simulink model "case6"  (R2024b)
settings: Solver=FixedStepAuto  StartTime=0  StopTime=1  FixedStep=1e-7  RelTol=1e-3
values from neighbouring files (symbols this model uses):
  SG_D_1_D = 0.01056    [IEEE9_case_parameters.m]    (also in case1_parameters.m; case2_parameters.m; case3_parameters.m; case4_parameters.m)
  SG_D_1_EnableSaturation = 0    [IEEE9_case_parameters.m]    (also in case1_parameters.m; case2_parameters.m; case3_parameters.m; case4_parameters.m)
  SG_D_1_f0 = 60    [IEEE9_case_parameters.m]    (also in case1_parameters.m; case2_parameters.m; case3_parameters.m; case4_parameters.m)
  SG_D_1_H = 7.5    [IEEE9_case_parameters.m]    (also in case1_parameters.m; case2_parameters.m; case3_parameters.m; case4_parameters.m)
  SG_D_1_K_A = 20    [IEEE9_case_parameters.m]    (also in case1_parameters.m; case2_parameters.m; case3_parameters.m; case4_parameters.m)
  SG_D_1_K_E = 1.000000e+1    (= 10)    [IEEE9_case_parameters.m]    (also in case1_parameters.m; case2_parameters.m; case3_parameters.m; case4_parameters.m)
  SG_D_1_K_F = 2.363    [IEEE9_case_parameters.m]    (also in case1_parameters.m; case2_parameters.m; case3_parameters.m; case4_parameters.m)
  SG_D_1_K_s = 0.5    [IEEE9_case_parameters.m]    (also in case1_parameters.m = 5; case2_parameters.m = 5; case3_parameters.m = 5; case4_parameters.m = 5)
  SG_D_1_R_a = 0.001088    [IEEE9_case_parameters.m]    (also in case1_parameters.m; case2_parameters.m; case3_parameters.m; case4_parameters.m)
  SG_D_1_S_A = 1    [IEEE9_case_parameters.m]    (also in case1_parameters.m; case2_parameters.m; case3_parameters.m; case4_parameters.m)
  SG_D_1_S_B = 0.103    [IEEE9_case_parameters.m]    (also in case1_parameters.m; case2_parameters.m; case3_parameters.m; case4_parameters.m)
  SG_D_1_S_N = 10.659857    [IEEE9_case_parameters.m]    (also in case1_parameters.m; case2_parameters.m; case3_parameters.m; case4_parameters.m)
  SG_D_1_SpeedPara = 200    [IEEE9_case_parameters.m]    (also in case1_parameters.m; case2_parameters.m; case3_parameters.m; case4_parameters.m)
  SG_D_1_T_0 = 0.720173    [IEEE9_case_parameters.m]    (also in case1_parameters.m = 0.755522; case2_parameters.m = 0.808931; case3_parameters.m = 0.869402; case4_parameters.m = 0.729316)
  SG_D_1_T_1 = 0.3    [IEEE9_case_parameters.m]    (also in case1_parameters.m; case2_parameters.m; case3_parameters.m; case4_parameters.m)
  SG_D_1_T_2 = 0.05    [IEEE9_case_parameters.m]    (also in case1_parameters.m; case2_parameters.m; case3_parameters.m; case4_parameters.m)
  SG_D_1_T_3 = 0.02    [IEEE9_case_parameters.m]    (also in case1_parameters.m; case2_parameters.m; case3_parameters.m; case4_parameters.m)
  SG_D_1_T_4 = 0.005    [IEEE9_case_parameters.m]    (also in case1_parameters.m; case2_parameters.m; case3_parameters.m; case4_parameters.m)
  SG_D_1_T_A = 0.02    [IEEE9_case_parameters.m]    (also in case1_parameters.m; case2_parameters.m; case3_parameters.m; case4_parameters.m)
  SG_D_1_T_dd = 8.000000e+0    (= 8)    [IEEE9_case_parameters.m]    (also in case1_parameters.m; case2_parameters.m; case3_parameters.m; case4_parameters.m)
  SG_D_1_T_ddd = 0.04    [IEEE9_case_parameters.m]    (also in case1_parameters.m; case2_parameters.m; case3_parameters.m; case4_parameters.m)
  SG_D_1_T_E = 0.314    [IEEE9_case_parameters.m]    (also in case1_parameters.m; case2_parameters.m; case3_parameters.m; case4_parameters.m)
  SG_D_1_T_F = 0.35    [IEEE9_case_parameters.m]    (also in case1_parameters.m; case2_parameters.m; case3_parameters.m; case4_parameters.m)
  SG_D_1_T_qd = 0.8    [IEEE9_case_parameters.m]    (also in case1_parameters.m; case2_parameters.m; case3_parameters.m; case4_parameters.m)
  SG_D_1_T_qdd = 0.02    [IEEE9_case_parameters.m]    (also in case1_parameters.m; case2_parameters.m; case3_parameters.m; case4_parameters.m)
  SG_D_1_T_speed = 0.1    [IEEE9_case_parameters.m]    (also in case1_parameters.m = 200; case2_parameters.m = 200; case3_parameters.m = 200; case4_parameters.m = 200)
  SG_D_1_T_w = 0.5    [IEEE9_case_parameters.m]    (also in case1_parameters.m; case2_parameters.m; case3_parameters.m; case4_parameters.m)
  SG_D_1_V_ref = 1.990276    [IEEE9_case_parameters.m]    (also in case1_parameters.m = 2.042296; case2_parameters.m = 2.051388; case3_parameters.m = 2.089584; case4_parameters.m = 2.01845)
  SG_D_1_w_ref = 376.991118    [IEEE9_case_parameters.m]    (also in case1_parameters.m; case2_parameters.m; case3_parameters.m; case4_parameters.m)
  SG_D_1_wb = 6.000000e+1    (= 60)    [IEEE9_case_parameters.m]    (also in case1_parameters.m; case2_parameters.m; case3_parameters.m; case4_parameters.m)
  SG_D_1_x_d = 1.9    [IEEE9_case_parameters.m]    (also in case1_parameters.m; case2_parameters.m; case3_parameters.m; case4_parameters.m)
  SG_D_1_x_dd = 0.302    [IEEE9_case_parameters.m]    (also in case1_parameters.m; case2_parameters.m; case3_parameters.m; case4_parameters.m)
  SG_D_1_x_ddd = 0.204    [IEEE9_case_parameters.m]    (also in case1_parameters.m; case2_parameters.m; case3_parameters.m; case4_parameters.m)
  SG_D_1_x_l = 0.05    [IEEE9_case_parameters.m]    (also in case1_parameters.m; case2_parameters.m; case3_parameters.m; case4_parameters.m)
  SG_D_1_x_q = 1.3    [IEEE9_case_parameters.m]    (also in case1_parameters.m; case2_parameters.m; case3_parameters.m; case4_parameters.m)
  SG_D_1_x_qd = 0.5    [IEEE9_case_parameters.m]    (also in case1_parameters.m; case2_parameters.m; case3_parameters.m; case4_parameters.m)
  SG_D_1_x_qdd = 0.3    [IEEE9_case_parameters.m]    (also in case1_parameters.m; case2_parameters.m; case3_parameters.m; case4_parameters.m)
  SG_D_2_D = 0.02    [IEEE9_case_parameters.m]    (also in case1_parameters.m; case2_parameters.m; case3_parameters.m; case4_parameters.m)
  SG_D_2_EnableSaturation = 0    [IEEE9_case_parameters.m]    (also in case1_parameters.m; case2_parameters.m; case3_parameters.m; case4_parameters.m)
  SG_D_2_f0 = 60    [IEEE9_case_parameters.m]    (also in case1_parameters.m; case2_parameters.m; case3_parameters.m; case4_parameters.m)
  SG_D_2_H = 8.000000e+0    (= 8)    [IEEE9_case_parameters.m]    (also in case1_parameters.m; case2_parameters.m; case3_parameters.m; case4_parameters.m)
  SG_D_2_K_A = 20    [IEEE9_case_parameters.m]    (also in case1_parameters.m; case2_parameters.m; case3_parameters.m; case4_parameters.m)
  SG_D_2_K_E = 1.000000e+1    (= 10)    [IEEE9_case_parameters.m]    (also in case1_parameters.m; case2_parameters.m; case3_parameters.m; case4_parameters.m)
  SG_D_2_K_F = 2.363    [IEEE9_case_parameters.m]    (also in case1_parameters.m; case2_parameters.m; case3_parameters.m; case4_parameters.m)
  SG_D_2_K_s = 0.5    [IEEE9_case_parameters.m]    (also in case1_parameters.m = 4; case2_parameters.m = 4; case3_parameters.m = 4; case4_parameters.m = 4)
  SG_D_2_R_a = 0.001088    [IEEE9_case_parameters.m]    (also in case1_parameters.m; case2_parameters.m; case3_parameters.m; case4_parameters.m)
  SG_D_2_S_A = 1    [IEEE9_case_parameters.m]    (also in case1_parameters.m; case2_parameters.m; case3_parameters.m; case4_parameters.m)
  SG_D_2_S_B = 0.103    [IEEE9_case_parameters.m]    (also in case1_parameters.m; case2_parameters.m; case3_parameters.m; case4_parameters.m)
  SG_D_2_S_N = 10.659857    [IEEE9_case_parameters.m]    (also in case1_parameters.m; case2_parameters.m; case3_parameters.m; case4_parameters.m)
  SG_D_2_SpeedPara = 200    [IEEE9_case_parameters.m]    (also in case1_parameters.m; case2_parameters.m; case3_parameters.m; case4_parameters.m)
  SG_D_2_T_0 = 1.632913    [IEEE9_case_parameters.m]    (also in case1_parameters.m = 1.632925; case2_parameters.m = 1.632915; case3_parameters.m = 1.632914; case4_parameters.m = 1.632927)
  SG_D_2_T_1 = 0.2    [IEEE9_case_parameters.m]    (also in case1_parameters.m; case2_parameters.m; case3_parameters.m; case4_parameters.m)
  SG_D_2_T_2 = 0.05    [IEEE9_case_parameters.m]    (also in case1_parameters.m; case2_parameters.m; case3_parameters.m; case4_parameters.m)
  SG_D_2_T_3 = 0.02    [IEEE9_case_parameters.m]    (also in case1_parameters.m; case2_parameters.m; case3_parameters.m; case4_parameters.m)
  SG_D_2_T_4 = 0.005    [IEEE9_case_parameters.m]    (also in case1_parameters.m; case2_parameters.m; case3_parameters.m; case4_parameters.m)
  SG_D_2_T_A = 0.02    [IEEE9_case_parameters.m]    (also in case1_parameters.m; case2_parameters.m; case3_parameters.m; case4_parameters.m)
  SG_D_2_T_dd = 7.9    [IEEE9_case_parameters.m]    (also in case1_parameters.m; case2_parameters.m; case3_parameters.m; case4_parameters.m)
  SG_D_2_T_ddd = 0.04    [IEEE9_case_parameters.m]    (also in case1_parameters.m; case2_parameters.m; case3_parameters.m; case4_parameters.m)
  SG_D_2_T_E = 0.314    [IEEE9_case_parameters.m]    (also in case1_parameters.m; case2_parameters.m; case3_parameters.m; case4_parameters.m)
  SG_D_2_T_F = 0.35    [IEEE9_case_parameters.m]    (also in case1_parameters.m; case2_parameters.m; case3_parameters.m; case4_parameters.m)
  SG_D_2_T_qd = 0.8    [IEEE9_case_parameters.m]    (also in case1_parameters.m; case2_parameters.m; case3_parameters.m; case4_parameters.m)
  SG_D_2_T_qdd = 0.015    [IEEE9_case_parameters.m]    (also in case1_parameters.m; case2_parameters.m; case3_parameters.m; case4_parameters.m)
  SG_D_2_T_speed = 0.1    [IEEE9_case_parameters.m]    (also in case1_parameters.m = 150; case2_parameters.m = 150; case3_parameters.m = 150; case4_parameters.m = 150)
  SG_D_2_T_w = 0.35    [IEEE9_case_parameters.m]    (also in case1_parameters.m; case2_parameters.m; case3_parameters.m; case4_parameters.m)
  SG_D_2_V_ref = 2.58547    [IEEE9_case_parameters.m]    (also in case1_parameters.m = 2.597896; case2_parameters.m = 2.587136; case3_parameters.m = 2.586042; case4_parameters.m = 2.599679)
  SG_D_2_w_ref = 376.991118    [IEEE9_case_parameters.m]    (also in case1_parameters.m; case2_parameters.m; case3_parameters.m; case4_parameters.m)
  SG_D_2_wb = 6.000000e+1    (= 60)    [IEEE9_case_parameters.m]    (also in case1_parameters.m; case2_parameters.m; case3_parameters.m; case4_parameters.m)
  SG_D_2_x_d = 1.8    [IEEE9_case_parameters.m]    (also in case1_parameters.m; case2_parameters.m; case3_parameters.m; case4_parameters.m)
  SG_D_2_x_dd = 0.302    [IEEE9_case_parameters.m]    (also in case1_parameters.m; case2_parameters.m; case3_parameters.m; case4_parameters.m)
  SG_D_2_x_ddd = 0.204    [IEEE9_case_parameters.m]    (also in case1_parameters.m; case2_parameters.m; case3_parameters.m; case4_parameters.m)
  SG_D_2_x_l = 0.05    [IEEE9_case_parameters.m]    (also in case1_parameters.m; case2_parameters.m; case3_parameters.m; case4_parameters.m)
  SG_D_2_x_q = 1.25    [IEEE9_case_parameters.m]    (also in case1_parameters.m; case2_parameters.m; case3_parameters.m; case4_parameters.m)
  SG_D_2_x_qd = 0.5    [IEEE9_case_parameters.m]    (also in case1_parameters.m; case2_parameters.m; case3_parameters.m; case4_parameters.m)
  SG_D_2_x_qdd = 0.3    [IEEE9_case_parameters.m]    (also in case1_parameters.m; case2_parameters.m; case3_parameters.m; case4_parameters.m)
  SG_D_3_D = 0.02    [IEEE9_case_parameters.m]    (also in case1_parameters.m; case2_parameters.m; case3_parameters.m; case4_parameters.m)
  SG_D_3_EnableSaturation = 0    [IEEE9_case_parameters.m]    (also in case1_parameters.m; case2_parameters.m; case3_parameters.m; case4_parameters.m)
  SG_D_3_f0 = 60    [IEEE9_case_parameters.m]    (also in case1_parameters.m; case2_parameters.m; case3_parameters.m; case4_parameters.m)
  SG_D_3_H = 7.7    [IEEE9_case_parameters.m]    (also in case1_parameters.m; case2_parameters.m; case3_parameters.m; case4_parameters.m)
  SG_D_3_K_A = 20    [IEEE9_case_parameters.m]    (also in case1_parameters.m; case2_parameters.m; case3_parameters.m; case4_parameters.m)
  SG_D_3_K_E = 1.000000e+1    (= 10)    [IEEE9_case_parameters.m]    (also in case1_parameters.m; case2_parameters.m; case3_parameters.m; case4_parameters.m)
  SG_D_3_K_F = 2.363    [IEEE9_case_parameters.m]    (also in case1_parameters.m; case2_parameters.m; case3_parameters.m; case4_parameters.m)
  SG_D_3_K_s = 0.2    [IEEE9_case_parameters.m]    (also in case1_parameters.m = 2; case2_parameters.m = 2; case3_parameters.m = 2; case4_parameters.m = 2)
  SG_D_3_R_a = 0.001088    [IEEE9_case_parameters.m]    (also in case1_parameters.m; case2_parameters.m; case3_parameters.m; case4_parameters.m)
  SG_D_3_S_A = 1    [IEEE9_case_parameters.m]    (also in case1_parameters.m; case2_parameters.m; case3_parameters.m; case4_parameters.m)
  SG_D_3_S_B = 0.103    [IEEE9_case_parameters.m]    (also in case1_parameters.m; case2_parameters.m; case3_parameters.m; case4_parameters.m)
  SG_D_3_S_N = 10.659857    [IEEE9_case_parameters.m]    (also in case1_parameters.m; case2_parameters.m; case3_parameters.m; case4_parameters.m)
  SG_D_3_SpeedPara = 200    [IEEE9_case_parameters.m]    (also in case1_parameters.m; case2_parameters.m; case3_parameters.m; case4_parameters.m)
  SG_D_3_T_0 = 0.850788    [IEEE9_case_parameters.m]    (also in case1_parameters.m = 0.850786; case2_parameters.m = 0.850787; case3_parameters.m; case4_parameters.m = 0.850786)
  SG_D_3_T_1 = 0.2    [IEEE9_case_parameters.m]    (also in case1_parameters.m; case2_parameters.m; case3_parameters.m; case4_parameters.m)
  SG_D_3_T_2 = 0.05    [IEEE9_case_parameters.m]    (also in case1_parameters.m; case2_parameters.m; case3_parameters.m; case4_parameters.m)
  SG_D_3_T_3 = 0.02    [IEEE9_case_parameters.m]    (also in case1_parameters.m; case2_parameters.m; case3_parameters.m; case4_parameters.m)
  SG_D_3_T_4 = 0.005    [IEEE9_case_parameters.m]    (also in case1_parameters.m; case2_parameters.m; case3_parameters.m; case4_parameters.m)
  SG_D_3_T_A = 0.02    [IEEE9_case_parameters.m]    (also in case1_parameters.m; case2_parameters.m; case3_parameters.m; case4_parameters.m)
  SG_D_3_T_dd = 8.1    [IEEE9_case_parameters.m]    (also in case1_parameters.m; case2_parameters.m; case3_parameters.m; case4_parameters.m)
  SG_D_3_T_ddd = 0.04    [IEEE9_case_parameters.m]    (also in case1_parameters.m; case2_parameters.m; case3_parameters.m; case4_parameters.m)
  SG_D_3_T_E = 0.314    [IEEE9_case_parameters.m]    (also in case1_parameters.m; case2_parameters.m; case3_parameters.m; case4_parameters.m)
  SG_D_3_T_F = 0.35    [IEEE9_case_parameters.m]    (also in case1_parameters.m; case2_parameters.m; case3_parameters.m; case4_parameters.m)
  SG_D_3_T_qd = 0.8    [IEEE9_case_parameters.m]    (also in case1_parameters.m; case2_parameters.m; case3_parameters.m; case4_parameters.m)
  SG_D_3_T_qdd = 0.015    [IEEE9_case_parameters.m]    (also in case1_parameters.m; case2_parameters.m; case3_parameters.m; case4_parameters.m)
  SG_D_3_T_speed = 0.1    [IEEE9_case_parameters.m]    (also in case1_parameters.m = 180; case2_parameters.m = 180; case3_parameters.m = 180; case4_parameters.m = 180)
  SG_D_3_T_w = 0.4    [IEEE9_case_parameters.m]    (also in case1_parameters.m; case2_parameters.m; case3_parameters.m; case4_parameters.m)
  SG_D_3_V_ref = 1.892727    [IEEE9_case_parameters.m]    (also in case1_parameters.m = 1.906439; case2_parameters.m = 1.895535; case3_parameters.m = 1.892105; case4_parameters.m = 1.906598)
  SG_D_3_w_ref = 376.991118    [IEEE9_case_parameters.m]    (also in case1_parameters.m; case2_parameters.m; case3_parameters.m; case4_parameters.m)
  SG_D_3_wb = 6.000000e+1    (= 60)    [IEEE9_case_parameters.m]    (also in case1_parameters.m; case2_parameters.m; case3_parameters.m; case4_parameters.m)
  SG_D_3_x_d = 1.85    [IEEE9_case_parameters.m]    (also in case1_parameters.m; case2_parameters.m; case3_parameters.m; case4_parameters.m)
  SG_D_3_x_dd = 0.302    [IEEE9_case_parameters.m]    (also in case1_parameters.m; case2_parameters.m; case3_parameters.m; case4_parameters.m)
  SG_D_3_x_ddd = 0.204    [IEEE9_case_parameters.m]    (also in case1_parameters.m; case2_parameters.m; case3_parameters.m; case4_parameters.m)
  SG_D_3_x_l = 0.05    [IEEE9_case_parameters.m]    (also in case1_parameters.m; case2_parameters.m; case3_parameters.m; case4_parameters.m)
  SG_D_3_x_q = 1.2    [IEEE9_case_parameters.m]    (also in case1_parameters.m; case2_parameters.m; case3_parameters.m; case4_parameters.m)
  SG_D_3_x_qd = 0.5    [IEEE9_case_parameters.m]    (also in case1_parameters.m; case2_parameters.m; case3_parameters.m; case4_parameters.m)
  SG_D_3_x_qdd = 0.3    [IEEE9_case_parameters.m]    (also in case1_parameters.m; case2_parameters.m; case3_parameters.m; case4_parameters.m)
(part 5 of 12)

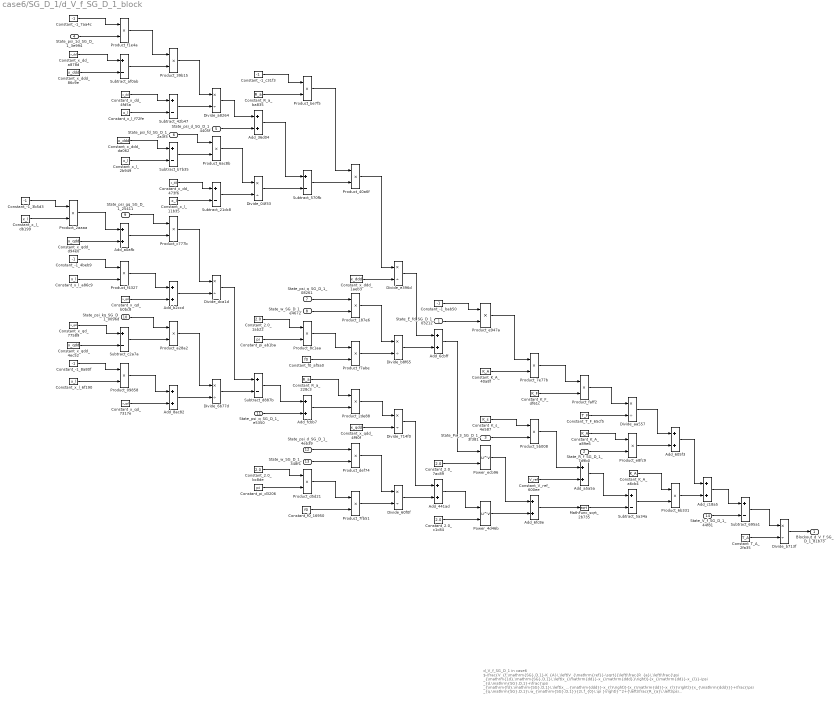
== system case6/SG_D_1/d_V_f_SG_D_1_block ==
  note: d_V_f_SG_D_1 in case6
      | $-\frac{V_{f,\mathrm{SG},D,1}-K_{A}\,\left(V_{\mathrm{ref}}-\sqrt{{\left(\frac{R_{a}\,\left(\frac{\psi _{\mathrm{1d},\mathrm{SG},D,1}\,\left(x_{\mathrm{dd}}-x_{\mathrm{ddd}}\right)}{x_{\mathrm{dd}}-x_{l}}-\psi _{d,\mathrm{SG},D,1}+\frac{\psi _{\mathrm{fd},\mathrm{SG},D,1}\,\left(x_{\mathrm{ddd}}-x_{l}\right)}{x_{\mathrm{dd}}-x_{l}}\right)}{x_{\mathrm{ddd}}}+\frac{\psi _{q,\mathrm{SG},D,1}\,w_{\mathrm{SG},D,1}}{2\,f_{0}\,\pi }\right)}^2+{\left(\frac{R_{a}\,\left(\psi _{q,\mathrm{SG},D,1}+\frac{\psi _{\mathrm{gq},\mathrm{SG},D,1}\,\left(x_{l}-x_{\mathrm{qdd}}\right)}{x_{l}-x_{\mathrm{qd}}}+\frac{\psi _{\mathrm{kq},\mathrm{SG},D,1}\,\left(x_{\mathrm{qd}}-x_{\mathrm{qdd}}\right)}{x_{l}-x_{\mathrm{qd}}}\right)}{x_{\mathrm{qdd}}}+\frac{\psi _{d,\mathrm{SG},D,1}\,w_{\mathrm{SG},D,1}}{2\,f_{0}\,\pi }\right)}^2}+K_{s}\,\mathrm{Px}_{3,\mathrm{SG},D,1}\right)-K_{A}\,R_{f,\mathrm{SG},D,1}+\frac{E_{\mathrm{fd},\mathrm{SG},D,1}\,K_{A}\,K_{F}}{T_{F}}}{T_{A}}$
      | Automatically generated on 2025-10-31 19:17:02 .
  State_E_fd_SG_D_1_03212 : Inport
  State_R_f_SG_D_1_7d9b0 : Inport  Port=2
  State_Px_3_SG_D_1_3f381 : Inport  Port=3
  State_psi_1d_SG_D_1_3e994 : Inport  Port=4
  State_psi_d_SG_D_1_4405f : Inport  Port=5
  State_psi_fd_SG_D_1_2a3f3 : Inport  Port=6
  State_psi_q_SG_D_1_08261 : Inport  Port=7
  State_w_SG_D_1_e4672 : Inport  Port=8
  State_psi_gq_SG_D_1_25411 : Inport  Port=9
  State_psi_kq_SG_D_1_0096d : Inport  Port=10
  State_psi_q_SG_D_1_e5350 : Inport  Port=11
  State_psi_d_SG_D_1_4eb39 : Inport  Port=12
  State_w_SG_D_1_348f1 : Inport  Port=13
  State_V_f_SG_D_1_44f81 : Inport  Port=14
  Add_36d04 : Sum
  Add_441ad : Sum
  Add_605f3 : Sum
  Add_6cbff : Sum
  Add_6fc8e : Sum
  Add_8ac82 : Sum
  Add_a0afb : Sum
  Add_a5a5a : Sum
  Add_b2ccd : Sum
  Add_c18a5 : Sum
  Add_fcbb7 : Sum
  Constant_-1_3b5d3 : Constant  Value=-1
  Constant_-1_4beb9 : Constant  Value=-1
  Constant_-1_7aa4c : Constant  Value=-1
  Constant_-1_8a80f : Constant  Value=-1
  Constant_-1_bab50 : Constant  Value=-1
  Constant_-1_c31f3 : Constant  Value=-1
  Constant_2.0_1ab22 : Constant  Value=2.0
  Constant_2.0_7ac89 : Constant  Value=2.0
  Constant_2.0_bc8de : Constant  Value=2.0
  Constant_2.0_c1c84 : Constant  Value=2.0
  Constant_K_A_40a8f : Constant  Value=K_A
  Constant_K_A_a6cb4 : Constant  Value=K_A
  Constant_K_A_a89e6 : Constant  Value=K_A
  Constant_K_F_df61c : Constant  Value=K_F
  Constant_K_s_4e587 : Constant  Value=K_s
  Constant_R_a_228c3 : Constant  Value=R_a
  Constant_R_a_ba835 : Constant  Value=R_a
  Constant_T_A_2fa35 : Constant  Value=T_A
  Constant_T_F_65cf5 : Constant  Value=T_F
  Constant_V_ref_600ee : Constant  Value=V_ref
  Constant_f0_16950 : Constant  Value=f0
  Constant_f0_af5a0 : Constant  Value=f0
  Constant_pi_ab1ba : Constant  Value=pi
  Constant_pi_d3206 : Constant  Value=pi
  Constant_x_dd_473f6 : Constant  Value=x_dd
  Constant_x_dd_4fd5a : Constant  Value=x_dd
  Constant_x_dd_a878d : Constant  Value=x_dd
  Constant_x_ddd_1aeb3 : Constant  Value=x_ddd
  Constant_x_ddd_86c9e : Constant  Value=x_ddd
  Constant_x_ddd_da062 : Constant  Value=x_ddd
  Constant_x_l_11b35 : Constant  Value=x_l
  Constant_x_l_2b949 : Constant  Value=x_l
  Constant_x_l_6f190 : Constant  Value=x_l
  Constant_x_l_a86c9 : Constant  Value=x_l
  Constant_x_l_db199 : Constant  Value=x_l
  Constant_x_l_f72fe : Constant  Value=x_l
  Constant_x_qd_7317e : Constant  Value=x_qd
  Constant_x_qd_77589 : Constant  Value=x_qd
  Constant_x_qd_b0bc8 : Constant  Value=x_qd
  Constant_x_qdd_4ec52 : Constant  Value=x_qdd
  Constant_x_qdd_4f90f : Constant  Value=x_qdd
  Constant_x_qdd_d94e0 : Constant  Value=x_qdd
  Divide_04f33 : Product  Inputs=*/
  Divide_60f0f : Product  Inputs=*/
  Divide_6b77d : Product  Inputs=*/
  Divide_714f0 : Product  Inputs=*/
  Divide_a8264 : Product  Inputs=*/
  Divide_aa557 : Product  Inputs=*/
  Divide_b713f : Product  Inputs=*/
  Divide_b8f65 : Product  Inputs=*/
  Divide_dca1d : Product  Inputs=*/
  Divide_e396d : Product  Inputs=*/
  MathFunc_sqrt_2b735 : Sqrt
  Power_4d46b : Math  Operator=pow
  Power_ecb96 : Math  Operator=pow
  Product_09858 : Product
  Product_187e6 : Product
  Product_2aaaa : Product
  Product_2de88 : Product
  Product_39b15 : Product
  Product_40a6f : Product
  Product_5b008 : Product
  Product_6ac8b : Product
  Product_6b331 : Product
  Product_7e77b : Product
  Product_7fb51 : Product
  Product_8c1aa : Product
  Product_a28a2 : Product
  Product_be7f5 : Product
  Product_c777b : Product
  Product_d5d21 : Product
  Product_def74 : Product
  Product_e8fc9 : Product
  Product_e947a : Product
  Product_f1e4a : Product
  Product_f4327 : Product
  Product_f7abe : Product
  Product_faff2 : Product
  Subtract_21dc8 : Sum  Inputs=+-
  Subtract_42b47 : Sum  Inputs=+-
  Subtract_570fb : Sum  Inputs=+-
  Subtract_5a34a : Sum  Inputs=+-
  Subtract_695a1 : Sum  Inputs=+-
  Subtract_af0ab : Sum  Inputs=+-
  Subtract_b7b35 : Sum  Inputs=+-
  Subtract_c2a7a : Sum  Inputs=+-
  Subtract_d887b : Sum  Inputs=+-
  Blockout_d_V_f_SG_D_1_81b73 : Outport
  wires:
  Constant_-1_8a80f/1 -> Product_09858/1
  Constant_-1_3b5d3/1 -> Product_2aaaa/1
  State_psi_d_SG_D_1_4eb39/1 -> Product_def74/1
  Constant_x_qd_7317e/1 -> Add_8ac82/2
  Constant_x_qdd_d94e0/1 -> Add_a0afb/2
  State_w_SG_D_1_348f1/1 -> Product_def74/2
  Constant_x_l_db199/1 -> Product_2aaaa/2
  Subtract_570fb/1 -> Product_40a6f/2
  Constant_x_l_6f190/1 -> Product_09858/2
  Constant_x_dd_a878d/1 -> Subtract_af0ab/1
  Constant_R_a_ba835/1 -> Product_be7f5/2
  Constant_-1_7aa4c/1 -> Product_f1e4a/1
  Divide_04f33/1 -> Subtract_570fb/2
  Constant_x_ddd_86c9e/1 -> Subtract_af0ab/2
  Add_8ac82/1 -> Divide_6b77d/2
  State_psi_1d_SG_D_1_3e994/1 -> Product_f1e4a/2
  Add_b2ccd/1 -> Divide_dca1d/2
  Subtract_c2a7a/1 -> Product_a28a2/2
  Product_faff2/1 -> Divide_aa557/1
  Product_8c1aa/1 -> Product_f7abe/1
  Product_2aaaa/1 -> Add_a0afb/1
  Constant_-1_4beb9/1 -> Product_f4327/1
  Constant_x_l_a86c9/1 -> Product_f4327/2
  Add_36d04/1 -> Subtract_570fb/1
  Constant_2.0_bc8de/1 -> Product_d5d21/1
  Constant_x_qd_77589/1 -> Subtract_c2a7a/1
  Product_f1e4a/1 -> Product_39b15/1
  Constant_pi_d3206/1 -> Product_d5d21/2
  Constant_x_qdd_4ec52/1 -> Subtract_c2a7a/2
  Subtract_af0ab/1 -> Product_39b15/2
  State_psi_q_SG_D_1_e5350/1 -> Add_fcbb7/2
  Constant_x_dd_4fd5a/1 -> Subtract_42b47/1
  Constant_x_l_f72fe/1 -> Subtract_42b47/2
  Constant_x_ddd_da062/1 -> Subtract_b7b35/1
  Constant_x_l_2b949/1 -> Subtract_b7b35/2
  State_psi_gq_SG_D_1_25411/1 -> Product_c777b/1
  Add_a0afb/1 -> Product_c777b/2
  Product_f4327/1 -> Add_b2ccd/1
  Constant_x_qd_b0bc8/1 -> Add_b2ccd/2
  Divide_a8264/1 -> Add_36d04/1
  Subtract_42b47/1 -> Divide_a8264/2
  State_psi_kq_SG_D_1_0096d/1 -> Product_a28a2/1
  Divide_b713f/1 -> Blockout_d_V_f_SG_D_1_81b73/1
  Product_09858/1 -> Add_8ac82/1
  Product_39b15/1 -> Divide_a8264/1
  State_psi_fd_SG_D_1_2a3f3/1 -> Product_6ac8b/1
  State_w_SG_D_1_e4672/1 -> Product_187e6/2
  Subtract_b7b35/1 -> Product_6ac8b/2
  Constant_x_dd_473f6/1 -> Subtract_21dc8/1
  Constant_x_l_11b35/1 -> Subtract_21dc8/2
  Product_c777b/1 -> Divide_dca1d/1
  Product_be7f5/1 -> Product_40a6f/1
  Product_a28a2/1 -> Divide_6b77d/1
  State_psi_d_SG_D_1_4405f/1 -> Add_36d04/2
  Product_6ac8b/1 -> Divide_04f33/1
  Subtract_21dc8/1 -> Divide_04f33/2
  Divide_dca1d/1 -> Subtract_d887b/1
  Divide_6b77d/1 -> Subtract_d887b/2
  Constant_-1_c31f3/1 -> Product_be7f5/1
  Constant_2.0_1ab22/1 -> Product_8c1aa/1
  Constant_pi_ab1ba/1 -> Product_8c1aa/2
  Subtract_d887b/1 -> Add_fcbb7/1
  State_psi_q_SG_D_1_08261/1 -> Product_187e6/1
  Constant_f0_af5a0/1 -> Product_f7abe/2
  Constant_R_a_228c3/1 -> Product_2de88/1
  Add_fcbb7/1 -> Product_2de88/2
  Product_d5d21/1 -> Product_7fb51/1
  Power_ecb96/1 -> Add_6fc8e/1
  Constant_f0_16950/1 -> Product_7fb51/2
  Product_40a6f/1 -> Divide_e396d/1
  Constant_x_ddd_1aeb3/1 -> Divide_e396d/2
  Product_187e6/1 -> Divide_b8f65/1
  Product_f7abe/1 -> Divide_b8f65/2
  Product_2de88/1 -> Divide_714f0/1
  Constant_x_qdd_4f90f/1 -> Divide_714f0/2
  Product_def74/1 -> Divide_60f0f/1
  Product_7fb51/1 -> Divide_60f0f/2
  Divide_e396d/1 -> Add_6cbff/1
  Divide_b8f65/1 -> Add_6cbff/2
  Divide_714f0/1 -> Add_441ad/1
  Divide_60f0f/1 -> Add_441ad/2
  Constant_-1_bab50/1 -> Product_e947a/1
  State_E_fd_SG_D_1_03212/1 -> Product_e947a/2
  Add_6cbff/1 -> Power_ecb96/1
  Constant_2.0_7ac89/1 -> Power_ecb96/2
  Add_441ad/1 -> Power_4d46b/1
  Constant_2.0_c1c84/1 -> Power_4d46b/2
  Product_e947a/1 -> Product_7e77b/1
  Constant_K_A_40a8f/1 -> Product_7e77b/2
  Constant_K_s_4e587/1 -> Product_5b008/1
  State_Px_3_SG_D_1_3f381/1 -> Product_5b008/2
  Power_4d46b/1 -> Add_6fc8e/2
  Divide_aa557/1 -> Add_605f3/1
  Product_7e77b/1 -> Product_faff2/1
  Constant_K_F_df61c/1 -> Product_faff2/2
  Product_5b008/1 -> Add_a5a5a/1
  Constant_V_ref_600ee/1 -> Add_a5a5a/2
  Add_6fc8e/1 -> MathFunc_sqrt_2b735/1
  Constant_T_F_65cf5/1 -> Divide_aa557/2
  Constant_K_A_a89e6/1 -> Product_e8fc9/1
  State_R_f_SG_D_1_7d9b0/1 -> Product_e8fc9/2
  Add_a5a5a/1 -> Subtract_5a34a/1
  MathFunc_sqrt_2b735/1 -> Subtract_5a34a/2
  Constant_T_A_2fa35/1 -> Divide_b713f/2
  Product_e8fc9/1 -> Add_605f3/2
  Constant_K_A_a6cb4/1 -> Product_6b331/1
  Subtract_5a34a/1 -> Product_6b331/2
  Add_605f3/1 -> Add_c18a5/1
  Product_6b331/1 -> Add_c18a5/2
  Add_c18a5/1 -> Subtract_695a1/1
  State_V_f_SG_D_1_44f81/1 -> Subtract_695a1/2
  Subtract_695a1/1 -> Divide_b713f/1

== system case6/SG_D_1/d_psi_1d_SG_D_1_block ==
  note: d_psi_1d_SG_D_1 in case6
      | $-\frac{\psi _{\mathrm{1d},\mathrm{SG},D,1}-\psi _{\mathrm{fd},\mathrm{SG},D,1}+\frac{\left(x_{\mathrm{dd}}-x_{l}\right)\,\left(\frac{\psi _{\mathrm{1d},\mathrm{SG},D,1}\,\left(x_{\mathrm{dd}}-x_{\mathrm{ddd}}\right)}{x_{\mathrm{dd}}-x_{l}}-\psi _{d,\mathrm{SG},D,1}+\frac{\psi _{\mathrm{fd},\mathrm{SG},D,1}\,\left(x_{\mathrm{ddd}}-x_{l}\right)}{x_{\mathrm{dd}}-x_{l}}\right)}{x_{\mathrm{ddd}}}}{T_{\mathrm{ddd}}}$
      | Automatically generated on 2025-10-31 19:16:38 .
  State_psi_1d_SG_D_1_4a698 : Inport
  State_psi_fd_SG_D_1_811e7 : Inport  Port=2
  State_psi_1d_SG_D_1_ea100 : Inport  Port=3
  State_psi_d_SG_D_1_f98fe : Inport  Port=4
  State_psi_fd_SG_D_1_382e7 : Inport  Port=5
  Add_2ab4c : Sum
  Add_6df2e : Sum
  Add_b1f1c : Sum
  Constant_-1_5b4ae : Constant  Value=-1
  Constant_-1_d8e8d : Constant  Value=-1
  Constant_T_ddd_942e3 : Constant  Value=T_ddd
  Constant_x_dd_465be : Constant  Value=x_dd
  Constant_x_dd_7c90c : Constant  Value=x_dd
  Constant_x_dd_cf83c : Constant  Value=x_dd
  Constant_x_dd_d9287 : Constant  Value=x_dd
  Constant_x_ddd_2eda3 : Constant  Value=x_ddd
  Constant_x_ddd_6c34b : Constant  Value=x_ddd
  Constant_x_ddd_8b575 : Constant  Value=x_ddd
  Constant_x_l_4735c : Constant  Value=x_l
  Constant_x_l_613d1 : Constant  Value=x_l
  Constant_x_l_9847b : Constant  Value=x_l
  Constant_x_l_a1b80 : Constant  Value=x_l
  Divide_32014 : Product  Inputs=*/
  Divide_46844 : Product  Inputs=*/
  Divide_bdf45 : Product  Inputs=*/
  Divide_ea900 : Product  Inputs=*/
  Product_727fc : Product
  Product_becc3 : Product
  Product_daa2b : Product
  Product_ee50c : Product
  Product_fa800 : Product
  Subtract_267db : Sum  Inputs=+-
  Subtract_53c96 : Sum  Inputs=+-
  Subtract_6044a : Sum  Inputs=+-
  Subtract_84949 : Sum  Inputs=+-
  Subtract_a7116 : Sum  Inputs=+-
  Subtract_d8e0a : Sum  Inputs=+-
  Blockout_d_psi_1d_SG_D_1_96faa : Outport
  wires:
  Product_becc3/1 -> Product_ee50c/1
  Constant_-1_d8e8d/1 -> Product_becc3/1
  Subtract_84949/1 -> Product_ee50c/2
  State_psi_1d_SG_D_1_ea100/1 -> Product_becc3/2
  Subtract_a7116/1 -> Product_727fc/1
  State_psi_d_SG_D_1_f98fe/1 -> Add_6df2e/2
  Constant_x_dd_7c90c/1 -> Subtract_d8e0a/1
  Constant_x_l_a1b80/1 -> Subtract_a7116/2
  Constant_x_dd_cf83c/1 -> Subtract_84949/1
  Subtract_53c96/1 -> Product_fa800/2
  Constant_x_l_613d1/1 -> Subtract_d8e0a/2
  Divide_bdf45/1 -> Subtract_267db/2
  Constant_x_ddd_6c34b/1 -> Subtract_84949/2
  Constant_x_ddd_8b575/1 -> Subtract_53c96/1
  Constant_x_l_9847b/1 -> Subtract_53c96/2
  Add_b1f1c/1 -> Add_2ab4c/1
  Product_ee50c/1 -> Divide_32014/1
  Divide_ea900/1 -> Add_2ab4c/2
  Subtract_d8e0a/1 -> Divide_32014/2
  State_psi_fd_SG_D_1_382e7/1 -> Product_fa800/1
  Constant_x_dd_465be/1 -> Subtract_6044a/1
  Constant_x_l_4735c/1 -> Subtract_6044a/2
  Constant_x_ddd_2eda3/1 -> Divide_ea900/2
  Subtract_267db/1 -> Product_727fc/2
  Divide_32014/1 -> Add_6df2e/1
  Product_fa800/1 -> Divide_bdf45/1
  Subtract_6044a/1 -> Divide_bdf45/2
  Product_727fc/1 -> Divide_ea900/1
  Constant_x_dd_d9287/1 -> Subtract_a7116/1
  Add_6df2e/1 -> Subtract_267db/1
  Constant_-1_5b4ae/1 -> Product_daa2b/1
  State_psi_1d_SG_D_1_4a698/1 -> Product_daa2b/2
  Product_daa2b/1 -> Add_b1f1c/1
  State_psi_fd_SG_D_1_811e7/1 -> Add_b1f1c/2
  Add_2ab4c/1 -> Divide_46844/1
  Constant_T_ddd_942e3/1 -> Divide_46844/2
  Divide_46844/1 -> Blockout_d_psi_1d_SG_D_1_96faa/1

== system case6/SG_D_1/d_psi_d_SG_D_1_block ==
  note: d_psi_d_SG_D_1 in case6
      | $2\,\pi \,f_{0}\,\left(v_{d,\mathrm{SG},D,1}\,\sin\left(\theta _{\mathrm{SG},D,1}\right)-v_{q,\mathrm{SG},D,1}\,\cos\left(\theta _{\mathrm{SG},D,1}\right)+\frac{R_{a}\,\left(\frac{\psi _{\mathrm{1d},\mathrm{SG},D,1}\,\left(x_{\mathrm{dd}}-x_{\mathrm{ddd}}\right)}{x_{\mathrm{dd}}-x_{l}}-\psi _{d,\mathrm{SG},D,1}+\frac{\psi _{\mathrm{fd},\mathrm{SG},D,1}\,\left(x_{\mathrm{ddd}}-x_{l}\right)}{x_{\mathrm{dd}}-x_{l}}\right)}{x_{\mathrm{ddd}}}+\frac{\psi _{q,\mathrm{SG},D,1}\,w_{\mathrm{SG},D,1}}{2\,f_{0}\,\pi }\right)$
      | Automatically generated on 2025-10-31 19:16:13 .
  State_psi_1d_SG_D_1_18a6b : Inport
  State_psi_d_SG_D_1_74963 : Inport  Port=2
  State_psi_fd_SG_D_1_3739e : Inport  Port=3
  Input_v_d_SG_D_1_e3573 : Inport  Port=4
  State_theta_SG_D_1_3bf9e : Inport  Port=5
  Input_v_q_SG_D_1_43df0 : Inport  Port=6
  State_theta_SG_D_1_fa062 : Inport  Port=7
  State_psi_q_SG_D_1_12fad : Inport  Port=8
  State_w_SG_D_1_b9cd2 : Inport  Port=9
  Add_86443 : Sum
  Add_d0eb0 : Sum
  Constant_-1_b3534 : Constant  Value=-1
  Constant_-2.0_95a0a : Constant  Value=-2.0
  Constant_2.0_c4a91 : Constant  Value=2.0
  Constant_R_a_96e3f : Constant  Value=R_a
  Constant_f0_67e99 : Constant  Value=f0
  Constant_f0_ec54c : Constant  Value=f0
  Constant_pi_4a159 : Constant  Value=pi
  Constant_pi_69152 : Constant  Value=pi
  Constant_x_dd_0af58 : Constant  Value=x_dd
  Constant_x_dd_6aa4d : Constant  Value=x_dd
  Constant_x_dd_a902f : Constant  Value=x_dd
  Constant_x_ddd_32ce8 : Constant  Value=x_ddd
  Constant_x_ddd_96fad : Constant  Value=x_ddd
  Constant_x_ddd_ad289 : Constant  Value=x_ddd
  Constant_x_l_9b6f0 : Constant  Value=x_l
  Constant_x_l_9fbb5 : Constant  Value=x_l
  Constant_x_l_c93d4 : Constant  Value=x_l
  Divide_1449b : Product  Inputs=*/
  Divide_4c3f6 : Product  Inputs=*/
  Divide_6dddb : Product  Inputs=*/
  Divide_7a8ae : Product  Inputs=*/
  MathFunc_cos_1f015 : Trigonometry  Operator=cos
  MathFunc_sin_bb303 : Trigonometry
  Product_08feb : Product
  Product_0d259 : Product
  Product_158af : Product
  Product_17e12 : Product
  Product_58d20 : Product
  Product_5c163 : Product
  Product_65432 : Product
  Product_a78fb : Product
  Product_b6fa4 : Product
  Product_c2953 : Product
  Product_e94e1 : Product
  Product_f2509 : Product
  Subtract_40edd : Sum  Inputs=+-
  Subtract_4533e : Sum  Inputs=+-
  Subtract_54690 : Sum  Inputs=+-
  Subtract_57dbb : Sum  Inputs=+-
  Subtract_73e0c : Sum  Inputs=+-
  Subtract_a5b0d : Sum  Inputs=+-
  Subtract_f2025 : Sum  Inputs=+-
  Blockout_d_psi_d_SG_D_1_543a6 : Outport
  wires:
  Add_d0eb0/1 -> Subtract_4533e/1
  Product_08feb/1 -> Divide_7a8ae/1
  Subtract_57dbb/1 -> Product_08feb/2
  Divide_7a8ae/1 -> Add_d0eb0/1
  Product_a78fb/1 -> Product_08feb/1
  Constant_x_ddd_32ce8/1 -> Subtract_57dbb/2
  Constant_x_dd_a902f/1 -> Subtract_57dbb/1
  State_psi_1d_SG_D_1_18a6b/1 -> Product_a78fb/2
  Constant_-1_b3534/1 -> Product_a78fb/1
  Product_e94e1/1 -> Divide_6dddb/1
  Constant_x_l_9fbb5/1 -> Subtract_a5b0d/2
  State_psi_d_SG_D_1_74963/1 -> Add_d0eb0/2
  Constant_x_dd_6aa4d/1 -> Subtract_a5b0d/1
  Constant_x_ddd_ad289/1 -> Subtract_40edd/1
  Constant_x_l_c93d4/1 -> Subtract_40edd/2
  Subtract_a5b0d/1 -> Divide_7a8ae/2
  State_psi_fd_SG_D_1_3739e/1 -> Product_e94e1/1
  Constant_x_ddd_96fad/1 -> Divide_4c3f6/2
  Subtract_40edd/1 -> Product_e94e1/2
  Product_58d20/1 -> Subtract_f2025/2
  Constant_x_dd_0af58/1 -> Subtract_54690/1
  Constant_x_l_9b6f0/1 -> Subtract_54690/2
  Subtract_54690/1 -> Divide_6dddb/2
  Divide_6dddb/1 -> Subtract_4533e/2
  Constant_R_a_96e3f/1 -> Product_b6fa4/1
  Subtract_4533e/1 -> Product_b6fa4/2
  MathFunc_cos_1f015/1 -> Product_65432/2
  State_theta_SG_D_1_3bf9e/1 -> MathFunc_sin_bb303/1
  Divide_4c3f6/1 -> Subtract_f2025/1
  Product_b6fa4/1 -> Divide_4c3f6/1
  MathFunc_sin_bb303/1 -> Product_58d20/2
  Input_v_d_SG_D_1_e3573/1 -> Product_58d20/1
  Product_c2953/1 -> Blockout_d_psi_d_SG_D_1_543a6/1
  Product_0d259/1 -> Product_c2953/1
  Product_f2509/1 -> Product_0d259/1
  State_theta_SG_D_1_fa062/1 -> MathFunc_cos_1f015/1
  Constant_2.0_c4a91/1 -> Product_5c163/1
  Constant_pi_69152/1 -> Product_5c163/2
  Input_v_q_SG_D_1_43df0/1 -> Product_65432/1
  Constant_f0_67e99/1 -> Product_0d259/2
  State_psi_q_SG_D_1_12fad/1 -> Product_17e12/1
  State_w_SG_D_1_b9cd2/1 -> Product_17e12/2
  Product_5c163/1 -> Product_158af/1
  Constant_pi_4a159/1 -> Product_f2509/2
  Constant_f0_ec54c/1 -> Product_158af/2
  Constant_-2.0_95a0a/1 -> Product_f2509/1
  Add_86443/1 -> Subtract_73e0c/1
  Subtract_f2025/1 -> Add_86443/1
  Product_65432/1 -> Add_86443/2
  Product_17e12/1 -> Divide_1449b/1
  Product_158af/1 -> Divide_1449b/2
  Divide_1449b/1 -> Subtract_73e0c/2
  Subtract_73e0c/1 -> Product_c2953/2

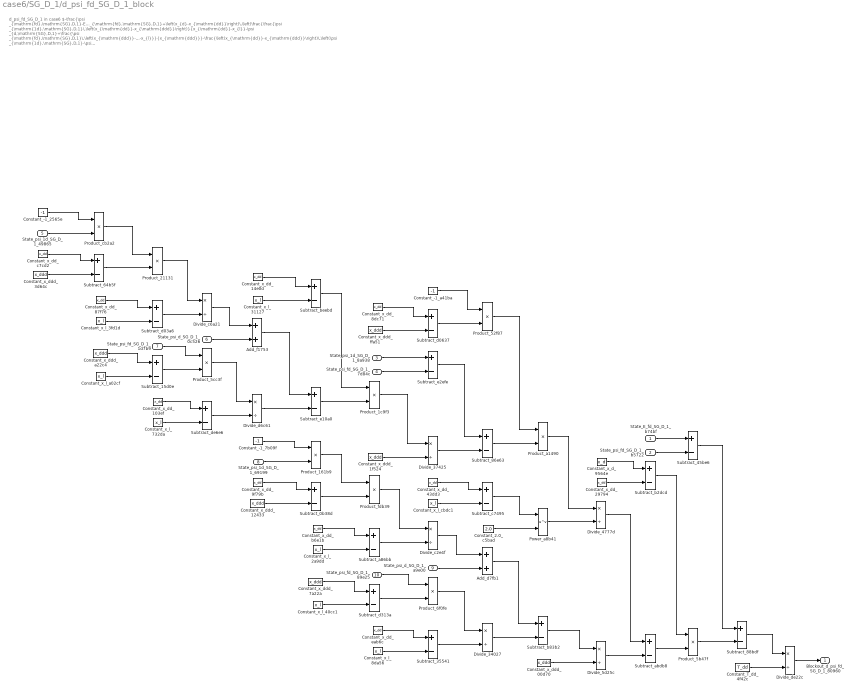
== system case6/SG_D_1/d_psi_fd_SG_D_1_block ==
  note: d_psi_fd_SG_D_1 in case6
      | $-\frac{\psi _{\mathrm{fd},\mathrm{SG},D,1}-E_{\mathrm{fd},\mathrm{SG},D,1}+\left(x_{d}-x_{\mathrm{dd}}\right)\,\left(\frac{\frac{\psi _{\mathrm{1d},\mathrm{SG},D,1}\,\left(x_{\mathrm{dd}}-x_{\mathrm{ddd}}\right)}{x_{\mathrm{dd}}-x_{l}}-\psi _{d,\mathrm{SG},D,1}+\frac{\psi _{\mathrm{fd},\mathrm{SG},D,1}\,\left(x_{\mathrm{ddd}}-x_{l}\right)}{x_{\mathrm{dd}}-x_{l}}}{x_{\mathrm{ddd}}}-\frac{\left(x_{\mathrm{dd}}-x_{\mathrm{ddd}}\right)\,\left(\psi _{\mathrm{1d},\mathrm{SG},D,1}-\psi _{\mathrm{fd},\mathrm{SG},D,1}+\frac{\left(x_{\mathrm{dd}}-x_{l}\right)\,\left(\frac{\psi _{\mathrm{1d},\mathrm{SG},D,1}\,\left(x_{\mathrm{dd}}-x_{\mathrm{ddd}}\right)}{x_{\mathrm{dd}}-x_{l}}-\psi _{d,\mathrm{SG},D,1}+\frac{\psi _{\mathrm{fd},\mathrm{SG},D,1}\,\left(x_{\mathrm{ddd}}-x_{l}\right)}{x_{\mathrm{dd}}-x_{l}}\right)}{x_{\mathrm{ddd}}}\right)}{{\left(x_{\mathrm{dd}}-x_{l}\right)}^2}\right)}{T_{\mathrm{dd}}}$
      | Automatically generated on 2025-10-31 19:16:35 .
  State_E_fd_SG_D_1_b74bf : Inport
  State_psi_fd_SG_D_1_b5722 : Inport  Port=2
  State_psi_1d_SG_D_1_8a938 : Inport  Port=3
  State_psi_fd_SG_D_1_7d84c : Inport  Port=4
  State_psi_1d_SG_D_1_49865 : Inport  Port=5
  State_psi_d_SG_D_1_0c526 : Inport  Port=6
  State_psi_fd_SG_D_1_1d7b9 : Inport  Port=7
  State_psi_1d_SG_D_1_69199 : Inport  Port=8
  State_psi_d_SG_D_1_a9e00 : Inport  Port=9
  State_psi_fd_SG_D_1_89e25 : Inport  Port=10
  Add_d7fb1 : Sum
  Add_f1753 : Sum
  Constant_-1_2565e : Constant  Value=-1
  Constant_-1_7b09f : Constant  Value=-1
  Constant_-1_a41ba : Constant  Value=-1
  Constant_2.0_c5bad : Constant  Value=2.0
  Constant_T_dd_4f42c : Constant  Value=T_dd
  Constant_x_d_9564e : Constant  Value=x_d
  Constant_x_dd_103ef : Constant  Value=x_dd
  Constant_x_dd_14e0d : Constant  Value=x_dd
  Constant_x_dd_29794 : Constant  Value=x_dd
  Constant_x_dd_43dd3 : Constant  Value=x_dd
  Constant_x_dd_87f76 : Constant  Value=x_dd
  Constant_x_dd_8dc71 : Constant  Value=x_dd
  Constant_x_dd_9f79b : Constant  Value=x_dd
  Constant_x_dd_b6e1b : Constant  Value=x_dd
  Constant_x_dd_c7cd2 : Constant  Value=x_dd
  Constant_x_dd_eab6c : Constant  Value=x_dd
  Constant_x_ddd_00d70 : Constant  Value=x_ddd
  Constant_x_ddd_12433 : Constant  Value=x_ddd
  Constant_x_ddd_1f524 : Constant  Value=x_ddd
  Constant_x_ddd_3d64c : Constant  Value=x_ddd
  Constant_x_ddd_7a22a : Constant  Value=x_ddd
  Constant_x_ddd_a22c4 : Constant  Value=x_ddd
  Constant_x_ddd_ffa51 : Constant  Value=x_ddd
  Constant_x_l_2a9dd : Constant  Value=x_l
  Constant_x_l_31127 : Constant  Value=x_l
  Constant_x_l_3fd1d : Constant  Value=x_l
  Constant_x_l_40cc1 : Constant  Value=x_l
  Constant_x_l_732da : Constant  Value=x_l
  Constant_x_l_8da56 : Constant  Value=x_l
  Constant_x_l_a02cf : Constant  Value=x_l
  Constant_x_l_cbdc1 : Constant  Value=x_l
  Divide_34027 : Product  Inputs=*/
  Divide_37425 : Product  Inputs=*/
  Divide_4777d : Product  Inputs=*/
  Divide_5d25c : Product  Inputs=*/
  Divide_c2e4f : Product  Inputs=*/
  Divide_c6a21 : Product  Inputs=*/
  Divide_d6c61 : Product  Inputs=*/
  Divide_de22c : Product  Inputs=*/
  Power_a8b41 : Math  Operator=pow
  Product_161b9 : Product
  Product_1c9f3 : Product
  Product_21131 : Product
  Product_52f87 : Product
  Product_5b47f : Product
  Product_5cc3f : Product
  Product_6f0fe : Product
  Product_a1490 : Product
  Product_cb2a2 : Product
  Product_fdb39 : Product
  Subtract_0b38d : Sum  Inputs=+-
  Subtract_15d0e : Sum  Inputs=+-
  Subtract_35541 : Sum  Inputs=+-
  Subtract_45be6 : Sum  Inputs=+-
  Subtract_64b5f : Sum  Inputs=+-
  Subtract_86e63 : Sum  Inputs=+-
  Subtract_88bdf : Sum  Inputs=+-
  Subtract_a86bb : Sum  Inputs=+-
  Subtract_abdb8 : Sum  Inputs=+-
  Subtract_b2dcd : Sum  Inputs=+-
  Subtract_b83b2 : Sum  Inputs=+-
  Subtract_beebd : Sum  Inputs=+-
  Subtract_c7495 : Sum  Inputs=+-
  Subtract_d03a6 : Sum  Inputs=+-
  Subtract_d0637 : Sum  Inputs=+-
  Subtract_d313a : Sum  Inputs=+-
  Subtract_de6e6 : Sum  Inputs=+-
  Subtract_e10a0 : Sum  Inputs=+-
  Subtract_e2efe : Sum  Inputs=+-
  Blockout_d_psi_fd_SG_D_1_80960 : Outport
  wires:
  State_psi_d_SG_D_1_0c526/1 -> Add_f1753/2
  Constant_x_dd_87f76/1 -> Subtract_d03a6/1
  Product_21131/1 -> Divide_c6a21/1
  Subtract_64b5f/1 -> Product_21131/2
  Subtract_e10a0/1 -> Product_1c9f3/2
  Product_cb2a2/1 -> Product_21131/1
  Constant_x_dd_c7cd2/1 -> Subtract_64b5f/1
  Constant_x_l_31127/1 -> Subtract_beebd/2
  Constant_-1_2565e/1 -> Product_cb2a2/1
  Subtract_beebd/1 -> Product_1c9f3/1
  Constant_x_l_3fd1d/1 -> Subtract_d03a6/2
  Constant_x_ddd_3d64c/1 -> Subtract_64b5f/2
  State_psi_1d_SG_D_1_49865/1 -> Product_cb2a2/2
  Constant_x_ddd_a22c4/1 -> Subtract_15d0e/1
  Constant_x_l_a02cf/1 -> Subtract_15d0e/2
  State_E_fd_SG_D_1_b74bf/1 -> Subtract_45be6/1
  Divide_c6a21/1 -> Add_f1753/1
  Subtract_d03a6/1 -> Divide_c6a21/2
  State_psi_fd_SG_D_1_1d7b9/1 -> Product_5cc3f/1
  Constant_x_ddd_1f524/1 -> Divide_37425/2
  Subtract_15d0e/1 -> Product_5cc3f/2
  Constant_x_dd_103ef/1 -> Subtract_de6e6/1
  Constant_x_dd_43dd3/1 -> Subtract_c7495/1
  State_psi_fd_SG_D_1_b5722/1 -> Subtract_45be6/2
  Constant_x_l_732da/1 -> Subtract_de6e6/2
  Product_5cc3f/1 -> Divide_d6c61/1
  Constant_-1_a41ba/1 -> Product_52f87/1
  Subtract_de6e6/1 -> Divide_d6c61/2
  Constant_x_dd_14e0d/1 -> Subtract_beebd/1
  Add_f1753/1 -> Subtract_e10a0/1
  Constant_x_l_cbdc1/1 -> Subtract_c7495/2
  Divide_d6c61/1 -> Subtract_e10a0/2
  Divide_4777d/1 -> Subtract_abdb8/1
  Constant_-1_7b09f/1 -> Product_161b9/1
  State_psi_1d_SG_D_1_69199/1 -> Product_161b9/2
  Constant_x_dd_9f79b/1 -> Subtract_0b38d/1
  Subtract_d0637/1 -> Product_52f87/2
  Constant_x_ddd_12433/1 -> Subtract_0b38d/2
  Product_161b9/1 -> Product_fdb39/1
  Constant_2.0_c5bad/1 -> Power_a8b41/2
  Product_fdb39/1 -> Divide_c2e4f/1
  Subtract_abdb8/1 -> Product_5b47f/2
  Subtract_0b38d/1 -> Product_fdb39/2
  State_psi_d_SG_D_1_a9e00/1 -> Add_d7fb1/2
  Constant_x_dd_b6e1b/1 -> Subtract_a86bb/1
  Constant_x_l_2a9dd/1 -> Subtract_a86bb/2
  Constant_x_dd_8dc71/1 -> Subtract_d0637/1
  Divide_37425/1 -> Subtract_86e63/2
  Constant_x_ddd_7a22a/1 -> Subtract_d313a/1
  Constant_x_ddd_ffa51/1 -> Subtract_d0637/2
  Constant_x_l_40cc1/1 -> Subtract_d313a/2
  Subtract_d313a/1 -> Product_6f0fe/2
  State_psi_1d_SG_D_1_8a938/1 -> Subtract_e2efe/1
  Product_6f0fe/1 -> Divide_34027/1
  State_psi_fd_SG_D_1_7d84c/1 -> Subtract_e2efe/2
  State_psi_fd_SG_D_1_89e25/1 -> Product_6f0fe/1
  Product_1c9f3/1 -> Divide_37425/1
  Divide_c2e4f/1 -> Add_d7fb1/1
  Subtract_a86bb/1 -> Divide_c2e4f/2
  Constant_x_dd_eab6c/1 -> Subtract_35541/1
  Constant_x_l_8da56/1 -> Subtract_35541/2
  Divide_34027/1 -> Subtract_b83b2/2
  Subtract_e2efe/1 -> Subtract_86e63/1
  Subtract_35541/1 -> Divide_34027/2
  Subtract_86e63/1 -> Product_a1490/2
  Product_52f87/1 -> Product_a1490/1
  Subtract_c7495/1 -> Power_a8b41/1
  Add_d7fb1/1 -> Subtract_b83b2/1
  Product_a1490/1 -> Divide_4777d/1
  Power_a8b41/1 -> Divide_4777d/2
  Subtract_b83b2/1 -> Divide_5d25c/1
  Constant_x_ddd_00d70/1 -> Divide_5d25c/2
  Constant_x_d_9564e/1 -> Subtract_b2dcd/1
  Constant_x_dd_29794/1 -> Subtract_b2dcd/2
  Divide_5d25c/1 -> Subtract_abdb8/2
  Subtract_b2dcd/1 -> Product_5b47f/1
  Subtract_45be6/1 -> Subtract_88bdf/1
  Product_5b47f/1 -> Subtract_88bdf/2
  Subtract_88bdf/1 -> Divide_de22c/1
  Constant_T_dd_4f42c/1 -> Divide_de22c/2
  Divide_de22c/1 -> Blockout_d_psi_fd_SG_D_1_80960/1

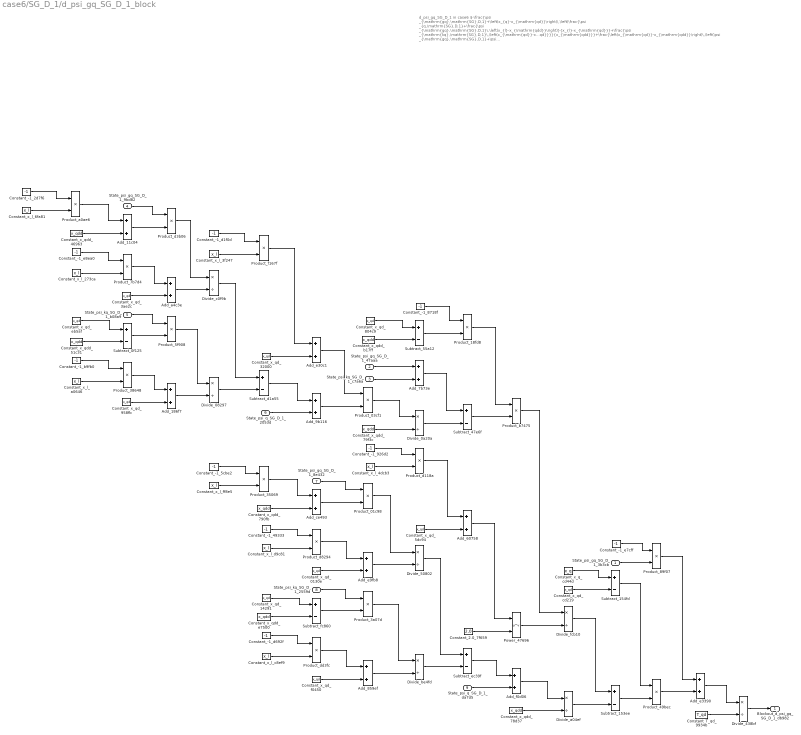
== system case6/SG_D_1/d_psi_gq_SG_D_1_block ==
  note: d_psi_gq_SG_D_1 in case6
      | $-\frac{\psi _{\mathrm{gq},\mathrm{SG},D,1}+\left(x_{q}-x_{\mathrm{qd}}\right)\,\left(\frac{\psi _{q,\mathrm{SG},D,1}+\frac{\psi _{\mathrm{gq},\mathrm{SG},D,1}\,\left(x_{l}-x_{\mathrm{qdd}}\right)}{x_{l}-x_{\mathrm{qd}}}+\frac{\psi _{\mathrm{kq},\mathrm{SG},D,1}\,\left(x_{\mathrm{qd}}-x_{\mathrm{qdd}}\right)}{x_{l}-x_{\mathrm{qd}}}}{x_{\mathrm{qdd}}}+\frac{\left(x_{\mathrm{qd}}-x_{\mathrm{qdd}}\right)\,\left(\psi _{\mathrm{gq},\mathrm{SG},D,1}+\psi _{\mathrm{kq},\mathrm{SG},D,1}+\frac{\left(x_{l}-x_{\mathrm{qd}}\right)\,\left(\psi _{q,\mathrm{SG},D,1}+\frac{\psi _{\mathrm{gq},\mathrm{SG},D,1}\,\left(x_{l}-x_{\mathrm{qdd}}\right)}{x_{l}-x_{\mathrm{qd}}}+\frac{\psi _{\mathrm{kq},\mathrm{SG},D,1}\,\left(x_{\mathrm{qd}}-x_{\mathrm{qdd}}\right)}{x_{l}-x_{\mathrm{qd}}}\right)}{x_{\mathrm{qdd}}}\right)}{{\left(x_{l}-x_{\mathrm{qd}}\right)}^2}\right)}{T_{\mathrm{qd}}}$
      | Automatically generated on 2025-10-31 19:16:44 .
  State_psi_gq_SG_D_1_3b3cb : Inport
  State_psi_gq_SG_D_1_47aaa : Inport  Port=2
  State_psi_kq_SG_D_1_c7a6a : Inport  Port=3
  State_psi_gq_SG_D_1_9bd82 : Inport  Port=4
  State_psi_kq_SG_D_1_b08a9 : Inport  Port=5
  State_psi_q_SG_D_1_2053d : Inport  Port=6
  State_psi_gq_SG_D_1_8e432 : Inport  Port=7
  State_psi_kq_SG_D_1_2559d : Inport  Port=8
  State_psi_q_SG_D_1_da7d5 : Inport  Port=9
  Add_11c04 : Sum
  Add_186f7 : Sum
  Add_60758 : Sum
  Add_7b73e : Sum
  Add_859ef : Sum
  Add_9b116 : Sum
  Add_a4c3e : Sum
  Add_ce493 : Sum
  Add_e30c1 : Sum
  Add_e3390 : Sum
  Add_e9fb8 : Sum
  Add_f0d06 : Sum
  Constant_-1_2d7f6 : Constant  Value=-1
  Constant_-1_49333 : Constant  Value=-1
  Constant_-1_5cbe2 : Constant  Value=-1
  Constant_-1_8718f : Constant  Value=-1
  Constant_-1_926d2 : Constant  Value=-1
  Constant_-1_b9fb0 : Constant  Value=-1
  Constant_-1_d1f0d : Constant  Value=-1
  Constant_-1_d692f : Constant  Value=-1
  Constant_-1_e7cff : Constant  Value=-1
  Constant_-1_e8ea0 : Constant  Value=-1
  Constant_2.0_7f659 : Constant  Value=2.0
  Constant_T_qd_9934b : Constant  Value=T_qd
  Constant_x_l_273ca : Constant  Value=x_l
  Constant_x_l_3f247 : Constant  Value=x_l
  Constant_x_l_4dcb3 : Constant  Value=x_l
  Constant_x_l_6fa81 : Constant  Value=x_l
  Constant_x_l_a0646 : Constant  Value=x_l
  Constant_x_l_c8ef9 : Constant  Value=x_l
  Constant_x_l_d9c81 : Constant  Value=x_l
  Constant_x_l_ff8e5 : Constant  Value=x_l
  Constant_x_q_cd44d : Constant  Value=x_q
  Constant_x_qd_0130e : Constant  Value=x_qd
  Constant_x_qd_14291 : Constant  Value=x_qd
  Constant_x_qd_32000 : Constant  Value=x_qd
  Constant_x_qd_3ae2c : Constant  Value=x_qd
  Constant_x_qd_5dc94 : Constant  Value=x_qd
  Constant_x_qd_804c9 : Constant  Value=x_qd
  Constant_x_qd_958fb : Constant  Value=x_qd
  Constant_x_qd_cd219 : Constant  Value=x_qd
  Constant_x_qd_eb5af : Constant  Value=x_qd
  Constant_x_qd_f0450 : Constant  Value=x_qd
  Constant_x_qdd_46963 : Constant  Value=x_qdd
  Constant_x_qdd_51c31 : Constant  Value=x_qdd
  Constant_x_qdd_78d37 : Constant  Value=x_qdd
  Constant_x_qdd_790fb : Constant  Value=x_qdd
  Constant_x_qdd_79f3c : Constant  Value=x_qdd
  Constant_x_qdd_b17ff : Constant  Value=x_qdd
  Constant_x_qdd_e7500 : Constant  Value=x_qdd
  Divide_08297 : Product  Inputs=*/
  Divide_0a20a : Product  Inputs=*/
  Divide_438bf : Product  Inputs=*/
  Divide_50802 : Product  Inputs=*/
  Divide_a04ef : Product  Inputs=*/
  Divide_be4fd : Product  Inputs=*/
  Divide_c0f9b : Product  Inputs=*/
  Divide_fcb10 : Product  Inputs=*/
  Power_47696 : Math  Operator=pow
  Product_01c98 : Product
  Product_03cf1 : Product
  Product_18fd8 : Product
  Product_35069 : Product
  Product_38648 : Product
  Product_3a07d : Product
  Product_49bec : Product
  Product_5f908 : Product
  Product_7b7d4 : Product
  Product_89f07 : Product
  Product_a0ae6 : Product
  Product_b7475 : Product
  Product_d118a : Product
  Product_d3b06 : Product
  Product_d8294 : Product
  Product_dd3fc : Product
  Product_f167f : Product
  Subtract_0f125 : Sum  Inputs=+-
  Subtract_153ee : Sum  Inputs=+-
  Subtract_154fd : Sum  Inputs=+-
  Subtract_47e6f : Sum  Inputs=+-
  Subtract_55a12 : Sum  Inputs=+-
  Subtract_d1a55 : Sum  Inputs=+-
  Subtract_ec39f : Sum  Inputs=+-
  Subtract_fc860 : Sum  Inputs=+-
  Blockout_d_psi_gq_SG_D_1_db982 : Outport
  wires:
  State_psi_gq_SG_D_1_9bd82/1 -> Product_d3b06/1
  Constant_-1_e8ea0/1 -> Product_7b7d4/1
  Divide_c0f9b/1 -> Subtract_d1a55/1
  Add_a4c3e/1 -> Divide_c0f9b/2
  Product_a0ae6/1 -> Add_11c04/1
  Constant_x_qd_32000/1 -> Add_e30c1/2
  Constant_-1_2d7f6/1 -> Product_a0ae6/1
  Constant_x_qdd_46963/1 -> Add_11c04/2
  Constant_x_l_273ca/1 -> Product_7b7d4/2
  Constant_x_l_6fa81/1 -> Product_a0ae6/2
  Constant_-1_b9fb0/1 -> Product_38648/1
  Constant_x_qd_eb5af/1 -> Subtract_0f125/1
  Constant_x_qdd_79f3c/1 -> Divide_0a20a/2
  Constant_x_l_a0646/1 -> Product_38648/2
  Constant_x_qdd_51c31/1 -> Subtract_0f125/2
  Subtract_d1a55/1 -> Add_9b116/1
  Add_11c04/1 -> Product_d3b06/2
  Product_d3b06/1 -> Divide_c0f9b/1
  Product_7b7d4/1 -> Add_a4c3e/1
  Constant_x_qd_3ae2c/1 -> Add_a4c3e/2
  State_psi_kq_SG_D_1_b08a9/1 -> Product_5f908/1
  Product_38648/1 -> Add_186f7/1
  Subtract_0f125/1 -> Product_5f908/2
  Constant_x_qd_958fb/1 -> Add_186f7/2
  Product_5f908/1 -> Divide_08297/1
  Add_186f7/1 -> Divide_08297/2
  Constant_-1_8718f/1 -> Product_18fd8/1
  Constant_-1_d1f0d/1 -> Product_f167f/1
  Add_e9fb8/1 -> Divide_50802/2
  Product_dd3fc/1 -> Add_859ef/1
  Subtract_fc860/1 -> Product_3a07d/2
  Constant_x_l_3f247/1 -> Product_f167f/2
  Divide_08297/1 -> Subtract_d1a55/2
  Subtract_154fd/1 -> Product_49bec/1
  Constant_-1_926d2/1 -> Product_d118a/1
  Constant_-1_5cbe2/1 -> Product_35069/1
  Constant_x_l_4dcb3/1 -> Product_d118a/2
  Constant_x_l_ff8e5/1 -> Product_35069/2
  Constant_x_qd_0130e/1 -> Add_e9fb8/2
  Product_f167f/1 -> Add_e30c1/1
  State_psi_q_SG_D_1_2053d/1 -> Add_9b116/2
  Product_35069/1 -> Add_ce493/1
  Constant_x_qdd_790fb/1 -> Add_ce493/2
  Constant_-1_49333/1 -> Product_d8294/1
  Constant_x_qd_f0450/1 -> Add_859ef/2
  Add_e30c1/1 -> Product_03cf1/1
  Constant_x_l_d9c81/1 -> Product_d8294/2
  Constant_-1_d692f/1 -> Product_dd3fc/1
  Constant_x_qd_14291/1 -> Subtract_fc860/1
  Product_03cf1/1 -> Divide_0a20a/1
  Constant_x_l_c8ef9/1 -> Product_dd3fc/2
  Divide_fcb10/1 -> Subtract_153ee/1
  Constant_x_qdd_e7500/1 -> Subtract_fc860/2
  Add_9b116/1 -> Product_03cf1/2
  State_psi_gq_SG_D_1_8e432/1 -> Product_01c98/1
  Add_ce493/1 -> Product_01c98/2
  Product_d8294/1 -> Add_e9fb8/1
  State_psi_kq_SG_D_1_2559d/1 -> Product_3a07d/1
  Add_859ef/1 -> Divide_be4fd/2
  State_psi_gq_SG_D_1_47aaa/1 -> Add_7b73e/1
  Constant_x_qd_804c9/1 -> Subtract_55a12/1
  Constant_x_qdd_b17ff/1 -> Subtract_55a12/2
  Product_3a07d/1 -> Divide_be4fd/1
  State_psi_kq_SG_D_1_c7a6a/1 -> Add_7b73e/2
  Product_01c98/1 -> Divide_50802/1
  Subtract_55a12/1 -> Product_18fd8/2
  Add_7b73e/1 -> Subtract_47e6f/1
  Divide_0a20a/1 -> Subtract_47e6f/2
  Product_d118a/1 -> Add_60758/1
  Constant_x_qd_5dc94/1 -> Add_60758/2
  Divide_50802/1 -> Subtract_ec39f/1
  Divide_be4fd/1 -> Subtract_ec39f/2
  Product_18fd8/1 -> Product_b7475/1
  Subtract_47e6f/1 -> Product_b7475/2
  Add_60758/1 -> Power_47696/1
  Constant_2.0_7f659/1 -> Power_47696/2
  Subtract_ec39f/1 -> Add_f0d06/1
  State_psi_q_SG_D_1_da7d5/1 -> Add_f0d06/2
  Product_b7475/1 -> Divide_fcb10/1
  Power_47696/1 -> Divide_fcb10/2
  Add_f0d06/1 -> Divide_a04ef/1
  Constant_x_qdd_78d37/1 -> Divide_a04ef/2
  Constant_x_q_cd44d/1 -> Subtract_154fd/1
  Constant_x_qd_cd219/1 -> Subtract_154fd/2
  Divide_a04ef/1 -> Subtract_153ee/2
  Constant_-1_e7cff/1 -> Product_89f07/1
  State_psi_gq_SG_D_1_3b3cb/1 -> Product_89f07/2
  Subtract_153ee/1 -> Product_49bec/2
  Product_89f07/1 -> Add_e3390/1
  Product_49bec/1 -> Add_e3390/2
  Add_e3390/1 -> Divide_438bf/1
  Constant_T_qd_9934b/1 -> Divide_438bf/2
  Divide_438bf/1 -> Blockout_d_psi_gq_SG_D_1_db982/1
